simulink model "ieee80211n"  (Simulink 6.0)
settings: Solver=VariableStepDiscrete  StartTime=0.0  StopTime=inf  RelTol=1e-3
PreLoadFcn:
  | load IEEE80211n_init;
values from neighbouring files (symbols this model uses):
  params =     [IEEE80211n_init.mat]    (also in IEEE80211n_settings.m = p)
undefined symbols (not defined in the file or in its folder): magnitude
libraries: commblkintrlv2 x196, dspsigops x143, simulink x136, commdigbbndam2 x98, dspmtrx3 x96, dspsigattribs x69, dspstat3 x38, commutil2 x32, commsequence2 x26, commcnvcod2 x10, dspindex x9, dspmlti3 x8
(part 11 of 12)

== system ieee80211n/training sequence4/Modulator1/Group into OFDM symbols ==
  in1 : Inport  Port=1  LatchInput=off
  in : Inport  Port=2  LatchInput=off
  Assemble Subcarriers : simulink/Math Operations/Matrix Concatenation  numInports=13  catMethod=Vertical
  DC value : Subsystem
      mask Display: disp('Zero DC')
  DC value1 : Subsystem
      mask Display: disp('Zeros, LB')
  DC value2 : Subsystem
      mask Display: disp('Zeros, UB')
  Gain : Gain  Gain=-1  SaturateOnIntegerOverflow=on
  Gain1 : Gain  Gain=-1  SaturateOnIntegerOverflow=on
  Select data blocks : S-Function  AncestorBlock=dspindex/Multiport Selector  FunctionName=sdspmultiportsel  Parameters=rowsOrCols, numOutports, flatIdxVect, flatLenVect, idxErrMode  mask(Multiport Selector){rowsOrCols=Rows, idxCellArray={1:5, 6:18, 19:24, 25:30, 31:43, 44:48}, idxErrMode=Clip Index}
      mask prompts: rowsOrCols "Select:"; idxCellArray "Indices to output:"; idxErrMode "Invalid index:"
      mask help: Output specified rows or columns to one or more output ports. The number of output ports is determined by the number of index vectors, each specified as a separate vector entry in a cell array. Indices are 1-based and need not be unique.
      mask init:
      | [numOutports, flatLenVect, flatIdxVect] = dspblkmultiportsel(idxCellArray);
      mask Help: web(dspbhelp);
      mask StyleString: popup(Rows|Columns),edit,popup(Clip Index|Clip and Warn|Generate Error)
      mask Display: disp(['Select\n' &1]);
  Select pilots : S-Function  AncestorBlock=dspindex/Multiport Selector  FunctionName=sdspmultiportsel  Parameters=rowsOrCols, numOutports, flatIdxVect, flatLenVect, idxErrMode  mask(Multiport Selector){rowsOrCols=Columns, idxCellArray={(1+params.OFDM_LSIG_SymPerFrame):(params.OFDM_LSIG_SymPerFrame+params.OFDM_HTSIG_SymPerFrame)}, idxErrMode=Clip Index}
      mask prompts: rowsOrCols "Select:"; idxCellArray "Indices to output:"; idxErrMode "Invalid index:"
      mask help: Output specified rows or columns to one or more output ports. The number of output ports is determined by the number of index vectors, each specified as a separate vector entry in a cell array. Indices are 1-based and need not be unique.
      mask init:
      | [numOutports, flatLenVect, flatIdxVect] = dspblkmultiportsel(idxCellArray);
      mask Help: web(dspbhelp);
      mask StyleString: popup(Rows|Columns),edit,popup(Clip Index|Clip and Warn|Generate Error)
      mask Display: disp(['Select\n' &1]);
  out : Outport
  wires:
  Select data blocks/1 -> Assemble Subcarriers/2
  Select data blocks/2 -> Assemble Subcarriers/4
  Select data blocks/3 -> Assemble Subcarriers/6
  Select data blocks/4 -> Assemble Subcarriers/8
  Select data blocks/5 -> Assemble Subcarriers/10
  Select data blocks/6 -> Assemble Subcarriers/12
  Gain/1 -> Assemble Subcarriers/11
  in1/1 -> Select pilots/1
  Assemble Subcarriers/1 -> out/1
  DC value/1(out) -> Assemble Subcarriers/7
  in/1 -> Select data blocks/1
  Select pilots/1 -> Gain1/1
  DC value1/1(out) -> Assemble Subcarriers/1
  DC value2/1(out) -> Assemble Subcarriers/13
  Gain1/1 -> Gain/1, Assemble Subcarriers/9, Assemble Subcarriers/5, Assemble Subcarriers/3

== system ieee80211n/training sequence4/Modulator1/Modulator 2 ==
  txdata : Inport  Port=1  LatchInput=off
  Convolutional Encoder1 : commcnvcod2/Convolutional Encoder  trellis=trellisStructure  reset=None
  Gain1 : Gain  SaturateOnIntegerOverflow=on
  General Block Interleaver : commblkintrlv2/General Block Interleaver  elements=interleaverElements
  Matrix Interleaver : commblkintrlv2/Matrix Interleaver  Nrows=interleaverRows  Ncols=interleaverCols
  P2 Puncture : commsequence2/Puncture  punctureVector=punctureVector
  Rectangular QAM Modulator Baseband : commdigbbndam2/Rectangular QAM Modulator Baseband  M=modOrder  InType=Bit  Enc=Gray  PowType=Average Power  MinDist=2  AvgPow=1  PeakPow=1  Ph=0  numSamp=1
  Zero Pad : dspsigops/Zero Pad  padSigAt=End  zpadAlong=Columns  padNumOutRowsSpecMethod=User-specified  numOutRows=bitsPerBlock  padNumOutColsSpecMethod=User-specified  numOutCols=1  trunc_flag=None
      settings: AttributesFormatString=\n
  txsig : Outport
  wires:
  Rectangular QAM Modulator Baseband/1 -> Gain1/1
  Gain1/1 -> txsig/1
  txdata/1 -> Zero Pad/1
  Convolutional Encoder1/1 -> P2 Puncture/1
  Matrix Interleaver/1 -> General Block Interleaver/1
  P2 Puncture/1 -> Matrix Interleaver/1
  General Block Interleaver/1 -> Rectangular QAM Modulator Baseband/1
  Zero Pad/1 -> Convolutional Encoder1/1

== system ieee80211n/training sequence4/Pilots/Unipolar to Bipolar Converter ==
  In1 : Inport  Port=1  LatchInput=off
  Constant : Constant  Orientation=up  Value=M-1
  Gain : Gain  Gain=2
  Polarity : Gain  Gain=pole
  Sum : Sum  Inputs=|+-  InputSameDT=on
  Out1 : Outport
  wires:
  Gain/1 -> Sum/1
  In1/1 -> Gain/1
  Sum/1 -> Polarity/1
  Constant/1 -> Sum/2
  Polarity/1 -> Out1/1

== system ieee80211n/MIMODetection/Channel Estimation/ChannelEst1/Channel estimates ==
  trn : Inport  Port=1  LatchInput=off
  in : Inport  Port=2  LatchInput=off
  Enable Averaging : MultiPortSwitch  Inputs=2  zeroidx=on  SaturateOnIntegerOverflow=on
  Enable Averaging1 : MultiPortSwitch  Inputs=2  zeroidx=on  SaturateOnIntegerOverflow=on
  Frame Status Conversion1 : dspsigattribs/Frame Status Conversion  growRefPort=off  outframe=Frame-based
  Mean : dspstat3/Mean  DialogController=dspDDGCreate  DialogControllerArgs=DataTag3  run=off  reset_popup=None  roundingMode=Floor  overflowMode=off
  Mean1 : dspstat3/Mean  DialogController=dspDDGCreate  DialogControllerArgs=DataTag4  run=off  reset_popup=None  roundingMode=Floor  overflowMode=off
  Nsts > 1 : Constant  Value=params.NSTS > 1
  One sym only (in) : S-Function  AncestorBlock=dspindex/Multiport Selector  FunctionName=sdspmultiportsel  Parameters=rowsOrCols, numOutports, flatIdxVect, flatLenVect, idxErrMode  mask(Multiport Selector){rowsOrCols=Rows, idxCellArray=1, idxErrMode=Clip Index}
      mask prompts: rowsOrCols "Select:"; idxCellArray "Indices to output:"; idxErrMode "Invalid index:"
      mask help: Output specified rows or columns to one or more output ports. The number of output ports is determined by the number of index vectors, each specified as a separate vector entry in a cell array. Indices are 1-based and need not be unique.
      mask init:
      | [numOutports, flatLenVect, flatIdxVect] = dspblkmultiportsel(idxCellArray);
      mask Help: web(dspbhelp);
      mask StyleString: popup(Rows|Columns),edit,popup(Clip Index|Clip and Warn|Generate Error)
      mask Display: disp(['Select\n' &1]);
  One sym only (trn) : S-Function  AncestorBlock=dspindex/Multiport Selector  FunctionName=sdspmultiportsel  Parameters=rowsOrCols, numOutports, flatIdxVect, flatLenVect, idxErrMode  mask(Multiport Selector){rowsOrCols=Rows, idxCellArray=1, idxErrMode=Clip Index}
      mask prompts: rowsOrCols "Select:"; idxCellArray "Indices to output:"; idxErrMode "Invalid index:"
      mask help: Output specified rows or columns to one or more output ports. The number of output ports is determined by the number of index vectors, each specified as a separate vector entry in a cell array. Indices are 1-based and need not be unique.
      mask init:
      | [numOutports, flatLenVect, flatIdxVect] = dspblkmultiportsel(idxCellArray);
      mask Help: web(dspbhelp);
      mask StyleString: popup(Rows|Columns),edit,popup(Clip Index|Clip and Warn|Generate Error)
      mask Display: disp(['Select\n' &1]);
  Product1 : Product  Inputs=**  SaturateOnIntegerOverflow=on
  Product3 : Product  Inputs=/*  SaturateOnIntegerOverflow=on
  Transpose : dspmtrx3/Transpose  Hermitian=off  overflowFlag=on
  Transpose1 : dspmtrx3/Transpose  Hermitian=off  overflowFlag=on
  Transpose2 : dspmtrx3/Transpose  Hermitian=off  overflowFlag=on
  ch est : Outport
  wires:
  trn/1 -> Transpose/1
  Mean/1 -> Enable Averaging/3
  Mean1/1 -> Enable Averaging1/3
  Product3/1 -> Frame Status Conversion1/1
  Transpose/1 -> Product1/1, Product1/2
  Frame Status Conversion1/1 -> Transpose1/1
  Transpose1/1 -> ch est/1
  Transpose2/1 -> Mean1/1, One sym only (in)/1
  Product1/1 -> Mean/1, One sym only (trn)/1
  in/1 -> Transpose2/1
  Enable Averaging/1 -> Product3/1
  Nsts > 1/1 -> Enable Averaging/1, Enable Averaging1/1
  One sym only (in)/1 -> Enable Averaging1/2
  Enable Averaging1/1 -> Product3/2
  One sym only (trn)/1 -> Enable Averaging/2

== system ieee80211n/MIMODetection/Channel Estimation/ChannelEst10/Channel estimates ==
  trn : Inport  Port=1  LatchInput=off
  in : Inport  Port=2  LatchInput=off
  Enable Averaging : MultiPortSwitch  Inputs=2  zeroidx=on  SaturateOnIntegerOverflow=on
  Enable Averaging1 : MultiPortSwitch  Inputs=2  zeroidx=on  SaturateOnIntegerOverflow=on
  Frame Status Conversion1 : dspsigattribs/Frame Status Conversion  growRefPort=off  outframe=Frame-based
  Mean2 : dspstat3/Mean  DialogController=dspDDGCreate  DialogControllerArgs=DataTag5  run=off  reset_popup=None  roundingMode=Floor  overflowMode=off
  Mean3 : dspstat3/Mean  DialogController=dspDDGCreate  DialogControllerArgs=DataTag6  run=off  reset_popup=None  roundingMode=Floor  overflowMode=off
  Nsts > 1 : Constant  Value=params.NSTS > 1
  One sym only (in) : S-Function  AncestorBlock=dspindex/Multiport Selector  FunctionName=sdspmultiportsel  Parameters=rowsOrCols, numOutports, flatIdxVect, flatLenVect, idxErrMode  mask(Multiport Selector){rowsOrCols=Rows, idxCellArray=1, idxErrMode=Clip Index}
      mask prompts: rowsOrCols "Select:"; idxCellArray "Indices to output:"; idxErrMode "Invalid index:"
      mask help: Output specified rows or columns to one or more output ports. The number of output ports is determined by the number of index vectors, each specified as a separate vector entry in a cell array. Indices are 1-based and need not be unique.
      mask init:
      | [numOutports, flatLenVect, flatIdxVect] = dspblkmultiportsel(idxCellArray);
      mask Help: web(dspbhelp);
      mask StyleString: popup(Rows|Columns),edit,popup(Clip Index|Clip and Warn|Generate Error)
      mask Display: disp(['Select\n' &1]);
  One sym only (trn) : S-Function  AncestorBlock=dspindex/Multiport Selector  FunctionName=sdspmultiportsel  Parameters=rowsOrCols, numOutports, flatIdxVect, flatLenVect, idxErrMode  mask(Multiport Selector){rowsOrCols=Rows, idxCellArray=1, idxErrMode=Clip Index}
      mask prompts: rowsOrCols "Select:"; idxCellArray "Indices to output:"; idxErrMode "Invalid index:"
      mask help: Output specified rows or columns to one or more output ports. The number of output ports is determined by the number of index vectors, each specified as a separate vector entry in a cell array. Indices are 1-based and need not be unique.
      mask init:
      | [numOutports, flatLenVect, flatIdxVect] = dspblkmultiportsel(idxCellArray);
      mask Help: web(dspbhelp);
      mask StyleString: popup(Rows|Columns),edit,popup(Clip Index|Clip and Warn|Generate Error)
      mask Display: disp(['Select\n' &1]);
  Product2 : Product  Inputs=**  SaturateOnIntegerOverflow=on
  Product4 : Product  Inputs=/*  SaturateOnIntegerOverflow=on
  Transpose : dspmtrx3/Transpose  Hermitian=off  overflowFlag=on
  Transpose1 : dspmtrx3/Transpose  Hermitian=off  overflowFlag=on
  Transpose2 : dspmtrx3/Transpose  Hermitian=off  overflowFlag=on
  ch est : Outport
  wires:
  trn/1 -> Transpose/1
  Product4/1 -> Frame Status Conversion1/1
  Frame Status Conversion1/1 -> Transpose1/1
  Transpose1/1 -> ch est/1
  in/1 -> Transpose2/1
  Mean2/1 -> Enable Averaging/3
  Mean3/1 -> Enable Averaging1/3
  Transpose/1 -> Product2/1, Product2/2
  Transpose2/1 -> Mean3/1, One sym only (in)/1
  Product2/1 -> Mean2/1, One sym only (trn)/1
  Enable Averaging/1 -> Product4/1
  Nsts > 1/1 -> Enable Averaging/1, Enable Averaging1/1
  One sym only (in)/1 -> Enable Averaging1/2
  Enable Averaging1/1 -> Product4/2
  One sym only (trn)/1 -> Enable Averaging/2

== system ieee80211n/MIMODetection/Channel Estimation/ChannelEst11/Channel estimates ==
  trn : Inport  Port=1  LatchInput=off
  in : Inport  Port=2  LatchInput=off
  Enable Averaging : MultiPortSwitch  Inputs=2  zeroidx=on  SaturateOnIntegerOverflow=on
  Enable Averaging1 : MultiPortSwitch  Inputs=2  zeroidx=on  SaturateOnIntegerOverflow=on
  Frame Status Conversion1 : dspsigattribs/Frame Status Conversion  growRefPort=off  outframe=Frame-based
  Mean2 : dspstat3/Mean  DialogController=dspDDGCreate  DialogControllerArgs=DataTag7  run=off  reset_popup=None  roundingMode=Floor  overflowMode=off
  Mean3 : dspstat3/Mean  DialogController=dspDDGCreate  DialogControllerArgs=DataTag8  run=off  reset_popup=None  roundingMode=Floor  overflowMode=off
  Nsts > 1 : Constant  Value=params.NSTS > 1
  One sym only (in) : S-Function  AncestorBlock=dspindex/Multiport Selector  FunctionName=sdspmultiportsel  Parameters=rowsOrCols, numOutports, flatIdxVect, flatLenVect, idxErrMode  mask(Multiport Selector){rowsOrCols=Rows, idxCellArray=1, idxErrMode=Clip Index}
      mask prompts: rowsOrCols "Select:"; idxCellArray "Indices to output:"; idxErrMode "Invalid index:"
      mask help: Output specified rows or columns to one or more output ports. The number of output ports is determined by the number of index vectors, each specified as a separate vector entry in a cell array. Indices are 1-based and need not be unique.
      mask init:
      | [numOutports, flatLenVect, flatIdxVect] = dspblkmultiportsel(idxCellArray);
      mask Help: web(dspbhelp);
      mask StyleString: popup(Rows|Columns),edit,popup(Clip Index|Clip and Warn|Generate Error)
      mask Display: disp(['Select\n' &1]);
  One sym only (trn) : S-Function  AncestorBlock=dspindex/Multiport Selector  FunctionName=sdspmultiportsel  Parameters=rowsOrCols, numOutports, flatIdxVect, flatLenVect, idxErrMode  mask(Multiport Selector){rowsOrCols=Rows, idxCellArray=1, idxErrMode=Clip Index}
      mask prompts: rowsOrCols "Select:"; idxCellArray "Indices to output:"; idxErrMode "Invalid index:"
      mask help: Output specified rows or columns to one or more output ports. The number of output ports is determined by the number of index vectors, each specified as a separate vector entry in a cell array. Indices are 1-based and need not be unique.
      mask init:
      | [numOutports, flatLenVect, flatIdxVect] = dspblkmultiportsel(idxCellArray);
      mask Help: web(dspbhelp);
      mask StyleString: popup(Rows|Columns),edit,popup(Clip Index|Clip and Warn|Generate Error)
      mask Display: disp(['Select\n' &1]);
  Product2 : Product  Inputs=**  SaturateOnIntegerOverflow=on
  Product4 : Product  Inputs=/*  SaturateOnIntegerOverflow=on
  Transpose : dspmtrx3/Transpose  Hermitian=off  overflowFlag=on
  Transpose1 : dspmtrx3/Transpose  Hermitian=off  overflowFlag=on
  Transpose2 : dspmtrx3/Transpose  Hermitian=off  overflowFlag=on
  ch est : Outport
  wires:
  trn/1 -> Transpose/1
  Product4/1 -> Frame Status Conversion1/1
  Frame Status Conversion1/1 -> Transpose1/1
  Transpose1/1 -> ch est/1
  in/1 -> Transpose2/1
  Mean2/1 -> Enable Averaging/3
  Mean3/1 -> Enable Averaging1/3
  Transpose/1 -> Product2/1, Product2/2
  Transpose2/1 -> Mean3/1, One sym only (in)/1
  Product2/1 -> Mean2/1, One sym only (trn)/1
  Enable Averaging/1 -> Product4/1
  Nsts > 1/1 -> Enable Averaging/1, Enable Averaging1/1
  One sym only (in)/1 -> Enable Averaging1/2
  Enable Averaging1/1 -> Product4/2
  One sym only (trn)/1 -> Enable Averaging/2

== system ieee80211n/MIMODetection/Channel Estimation/ChannelEst12/Channel estimates ==
  trn : Inport  Port=1  LatchInput=off
  in : Inport  Port=2  LatchInput=off
  Enable Averaging : MultiPortSwitch  Inputs=2  zeroidx=on  SaturateOnIntegerOverflow=on
  Enable Averaging1 : MultiPortSwitch  Inputs=2  zeroidx=on  SaturateOnIntegerOverflow=on
  Frame Status Conversion1 : dspsigattribs/Frame Status Conversion  growRefPort=off  outframe=Frame-based
  Mean2 : dspstat3/Mean  DialogController=dspDDGCreate  DialogControllerArgs=DataTag9  run=off  reset_popup=None  roundingMode=Floor  overflowMode=off
  Mean3 : dspstat3/Mean  DialogController=dspDDGCreate  DialogControllerArgs=DataTag10  run=off  reset_popup=None  roundingMode=Floor  overflowMode=off
  Nsts > 1 : Constant  Value=params.NSTS > 1
  One sym only (in) : S-Function  AncestorBlock=dspindex/Multiport Selector  FunctionName=sdspmultiportsel  Parameters=rowsOrCols, numOutports, flatIdxVect, flatLenVect, idxErrMode  mask(Multiport Selector){rowsOrCols=Rows, idxCellArray=1, idxErrMode=Clip Index}
      mask prompts: rowsOrCols "Select:"; idxCellArray "Indices to output:"; idxErrMode "Invalid index:"
      mask help: Output specified rows or columns to one or more output ports. The number of output ports is determined by the number of index vectors, each specified as a separate vector entry in a cell array. Indices are 1-based and need not be unique.
      mask init:
      | [numOutports, flatLenVect, flatIdxVect] = dspblkmultiportsel(idxCellArray);
      mask Help: web(dspbhelp);
      mask StyleString: popup(Rows|Columns),edit,popup(Clip Index|Clip and Warn|Generate Error)
      mask Display: disp(['Select\n' &1]);
  One sym only (trn) : S-Function  AncestorBlock=dspindex/Multiport Selector  FunctionName=sdspmultiportsel  Parameters=rowsOrCols, numOutports, flatIdxVect, flatLenVect, idxErrMode  mask(Multiport Selector){rowsOrCols=Rows, idxCellArray=1, idxErrMode=Clip Index}
      mask prompts: rowsOrCols "Select:"; idxCellArray "Indices to output:"; idxErrMode "Invalid index:"
      mask help: Output specified rows or columns to one or more output ports. The number of output ports is determined by the number of index vectors, each specified as a separate vector entry in a cell array. Indices are 1-based and need not be unique.
      mask init:
      | [numOutports, flatLenVect, flatIdxVect] = dspblkmultiportsel(idxCellArray);
      mask Help: web(dspbhelp);
      mask StyleString: popup(Rows|Columns),edit,popup(Clip Index|Clip and Warn|Generate Error)
      mask Display: disp(['Select\n' &1]);
  Product2 : Product  Inputs=**  SaturateOnIntegerOverflow=on
  Product4 : Product  Inputs=/*  SaturateOnIntegerOverflow=on
  Transpose : dspmtrx3/Transpose  Hermitian=off  overflowFlag=on
  Transpose1 : dspmtrx3/Transpose  Hermitian=off  overflowFlag=on
  Transpose2 : dspmtrx3/Transpose  Hermitian=off  overflowFlag=on
  ch est : Outport
  wires:
  trn/1 -> Transpose/1
  Product4/1 -> Frame Status Conversion1/1
  Frame Status Conversion1/1 -> Transpose1/1
  Transpose1/1 -> ch est/1
  in/1 -> Transpose2/1
  Mean2/1 -> Enable Averaging/3
  Mean3/1 -> Enable Averaging1/3
  Transpose/1 -> Product2/1, Product2/2
  Transpose2/1 -> Mean3/1, One sym only (in)/1
  Product2/1 -> Mean2/1, One sym only (trn)/1
  Enable Averaging/1 -> Product4/1
  Nsts > 1/1 -> Enable Averaging/1, Enable Averaging1/1
  One sym only (in)/1 -> Enable Averaging1/2
  Enable Averaging1/1 -> Product4/2
  One sym only (trn)/1 -> Enable Averaging/2

== system ieee80211n/MIMODetection/Channel Estimation/ChannelEst13/Channel estimates ==
  trn : Inport  Port=1  LatchInput=off
  in : Inport  Port=2  LatchInput=off
  Enable Averaging : MultiPortSwitch  Inputs=2  zeroidx=on  SaturateOnIntegerOverflow=on
  Enable Averaging1 : MultiPortSwitch  Inputs=2  zeroidx=on  SaturateOnIntegerOverflow=on
  Frame Status Conversion1 : dspsigattribs/Frame Status Conversion  growRefPort=off  outframe=Frame-based
  Mean2 : dspstat3/Mean  DialogController=dspDDGCreate  DialogControllerArgs=DataTag11  run=off  reset_popup=None  roundingMode=Floor  overflowMode=off
  Mean3 : dspstat3/Mean  DialogController=dspDDGCreate  DialogControllerArgs=DataTag12  run=off  reset_popup=None  roundingMode=Floor  overflowMode=off
  Nsts > 1 : Constant  Value=params.NSTS > 1
  One sym only (in) : S-Function  AncestorBlock=dspindex/Multiport Selector  FunctionName=sdspmultiportsel  Parameters=rowsOrCols, numOutports, flatIdxVect, flatLenVect, idxErrMode  mask(Multiport Selector){rowsOrCols=Rows, idxCellArray=1, idxErrMode=Clip Index}
      mask prompts: rowsOrCols "Select:"; idxCellArray "Indices to output:"; idxErrMode "Invalid index:"
      mask help: Output specified rows or columns to one or more output ports. The number of output ports is determined by the number of index vectors, each specified as a separate vector entry in a cell array. Indices are 1-based and need not be unique.
      mask init:
      | [numOutports, flatLenVect, flatIdxVect] = dspblkmultiportsel(idxCellArray);
      mask Help: web(dspbhelp);
      mask StyleString: popup(Rows|Columns),edit,popup(Clip Index|Clip and Warn|Generate Error)
      mask Display: disp(['Select\n' &1]);
  One sym only (trn) : S-Function  AncestorBlock=dspindex/Multiport Selector  FunctionName=sdspmultiportsel  Parameters=rowsOrCols, numOutports, flatIdxVect, flatLenVect, idxErrMode  mask(Multiport Selector){rowsOrCols=Rows, idxCellArray=1, idxErrMode=Clip Index}
      mask prompts: rowsOrCols "Select:"; idxCellArray "Indices to output:"; idxErrMode "Invalid index:"
      mask help: Output specified rows or columns to one or more output ports. The number of output ports is determined by the number of index vectors, each specified as a separate vector entry in a cell array. Indices are 1-based and need not be unique.
      mask init:
      | [numOutports, flatLenVect, flatIdxVect] = dspblkmultiportsel(idxCellArray);
      mask Help: web(dspbhelp);
      mask StyleString: popup(Rows|Columns),edit,popup(Clip Index|Clip and Warn|Generate Error)
      mask Display: disp(['Select\n' &1]);
  Product2 : Product  Inputs=**  SaturateOnIntegerOverflow=on
  Product4 : Product  Inputs=/*  SaturateOnIntegerOverflow=on
  Transpose : dspmtrx3/Transpose  Hermitian=off  overflowFlag=on
  Transpose1 : dspmtrx3/Transpose  Hermitian=off  overflowFlag=on
  Transpose2 : dspmtrx3/Transpose  Hermitian=off  overflowFlag=on
  ch est : Outport
  wires:
  trn/1 -> Transpose/1
  Product4/1 -> Frame Status Conversion1/1
  Frame Status Conversion1/1 -> Transpose1/1
  Transpose1/1 -> ch est/1
  in/1 -> Transpose2/1
  Mean2/1 -> Enable Averaging/3
  Mean3/1 -> Enable Averaging1/3
  Transpose/1 -> Product2/1, Product2/2
  Transpose2/1 -> Mean3/1, One sym only (in)/1
  Product2/1 -> Mean2/1, One sym only (trn)/1
  Enable Averaging/1 -> Product4/1
  Nsts > 1/1 -> Enable Averaging/1, Enable Averaging1/1
  One sym only (in)/1 -> Enable Averaging1/2
  Enable Averaging1/1 -> Product4/2
  One sym only (trn)/1 -> Enable Averaging/2

== system ieee80211n/MIMODetection/Channel Estimation/ChannelEst14/Channel estimates ==
  trn : Inport  Port=1  LatchInput=off
  in : Inport  Port=2  LatchInput=off
  Enable Averaging : MultiPortSwitch  Inputs=2  zeroidx=on  SaturateOnIntegerOverflow=on
  Enable Averaging1 : MultiPortSwitch  Inputs=2  zeroidx=on  SaturateOnIntegerOverflow=on
  Frame Status Conversion1 : dspsigattribs/Frame Status Conversion  growRefPort=off  outframe=Frame-based
  Mean2 : dspstat3/Mean  DialogController=dspDDGCreate  DialogControllerArgs=DataTag13  run=off  reset_popup=None  roundingMode=Floor  overflowMode=off
  Mean3 : dspstat3/Mean  DialogController=dspDDGCreate  DialogControllerArgs=DataTag14  run=off  reset_popup=None  roundingMode=Floor  overflowMode=off
  Nsts > 1 : Constant  Value=params.NSTS > 1
  One sym only (in) : S-Function  AncestorBlock=dspindex/Multiport Selector  FunctionName=sdspmultiportsel  Parameters=rowsOrCols, numOutports, flatIdxVect, flatLenVect, idxErrMode  mask(Multiport Selector){rowsOrCols=Rows, idxCellArray=1, idxErrMode=Clip Index}
      mask prompts: rowsOrCols "Select:"; idxCellArray "Indices to output:"; idxErrMode "Invalid index:"
      mask help: Output specified rows or columns to one or more output ports. The number of output ports is determined by the number of index vectors, each specified as a separate vector entry in a cell array. Indices are 1-based and need not be unique.
      mask init:
      | [numOutports, flatLenVect, flatIdxVect] = dspblkmultiportsel(idxCellArray);
      mask Help: web(dspbhelp);
      mask StyleString: popup(Rows|Columns),edit,popup(Clip Index|Clip and Warn|Generate Error)
      mask Display: disp(['Select\n' &1]);
  One sym only (trn) : S-Function  AncestorBlock=dspindex/Multiport Selector  FunctionName=sdspmultiportsel  Parameters=rowsOrCols, numOutports, flatIdxVect, flatLenVect, idxErrMode  mask(Multiport Selector){rowsOrCols=Rows, idxCellArray=1, idxErrMode=Clip Index}
      mask prompts: rowsOrCols "Select:"; idxCellArray "Indices to output:"; idxErrMode "Invalid index:"
      mask help: Output specified rows or columns to one or more output ports. The number of output ports is determined by the number of index vectors, each specified as a separate vector entry in a cell array. Indices are 1-based and need not be unique.
      mask init:
      | [numOutports, flatLenVect, flatIdxVect] = dspblkmultiportsel(idxCellArray);
      mask Help: web(dspbhelp);
      mask StyleString: popup(Rows|Columns),edit,popup(Clip Index|Clip and Warn|Generate Error)
      mask Display: disp(['Select\n' &1]);
  Product2 : Product  Inputs=**  SaturateOnIntegerOverflow=on
  Product4 : Product  Inputs=/*  SaturateOnIntegerOverflow=on
  Transpose : dspmtrx3/Transpose  Hermitian=off  overflowFlag=on
  Transpose1 : dspmtrx3/Transpose  Hermitian=off  overflowFlag=on
  Transpose2 : dspmtrx3/Transpose  Hermitian=off  overflowFlag=on
  ch est : Outport
  wires:
  trn/1 -> Transpose/1
  Product4/1 -> Frame Status Conversion1/1
  Frame Status Conversion1/1 -> Transpose1/1
  Transpose1/1 -> ch est/1
  in/1 -> Transpose2/1
  Mean2/1 -> Enable Averaging/3
  Mean3/1 -> Enable Averaging1/3
  Transpose/1 -> Product2/1, Product2/2
  Transpose2/1 -> Mean3/1, One sym only (in)/1
  Product2/1 -> Mean2/1, One sym only (trn)/1
  Enable Averaging/1 -> Product4/1
  Nsts > 1/1 -> Enable Averaging/1, Enable Averaging1/1
  One sym only (in)/1 -> Enable Averaging1/2
  Enable Averaging1/1 -> Product4/2
  One sym only (trn)/1 -> Enable Averaging/2

== system ieee80211n/MIMODetection/Channel Estimation/ChannelEst15/Channel estimates ==
  trn : Inport  Port=1  LatchInput=off
  in : Inport  Port=2  LatchInput=off
  Enable Averaging : MultiPortSwitch  Inputs=2  zeroidx=on  SaturateOnIntegerOverflow=on
  Enable Averaging1 : MultiPortSwitch  Inputs=2  zeroidx=on  SaturateOnIntegerOverflow=on
  Frame Status Conversion1 : dspsigattribs/Frame Status Conversion  growRefPort=off  outframe=Frame-based
  Mean2 : dspstat3/Mean  DialogController=dspDDGCreate  DialogControllerArgs=DataTag15  run=off  reset_popup=None  roundingMode=Floor  overflowMode=off
  Mean3 : dspstat3/Mean  DialogController=dspDDGCreate  DialogControllerArgs=DataTag16  run=off  reset_popup=None  roundingMode=Floor  overflowMode=off
  Nsts > 1 : Constant  Value=params.NSTS > 1
  One sym only (in) : S-Function  AncestorBlock=dspindex/Multiport Selector  FunctionName=sdspmultiportsel  Parameters=rowsOrCols, numOutports, flatIdxVect, flatLenVect, idxErrMode  mask(Multiport Selector){rowsOrCols=Rows, idxCellArray=1, idxErrMode=Clip Index}
      mask prompts: rowsOrCols "Select:"; idxCellArray "Indices to output:"; idxErrMode "Invalid index:"
      mask help: Output specified rows or columns to one or more output ports. The number of output ports is determined by the number of index vectors, each specified as a separate vector entry in a cell array. Indices are 1-based and need not be unique.
      mask init:
      | [numOutports, flatLenVect, flatIdxVect] = dspblkmultiportsel(idxCellArray);
      mask Help: web(dspbhelp);
      mask StyleString: popup(Rows|Columns),edit,popup(Clip Index|Clip and Warn|Generate Error)
      mask Display: disp(['Select\n' &1]);
  One sym only (trn) : S-Function  AncestorBlock=dspindex/Multiport Selector  FunctionName=sdspmultiportsel  Parameters=rowsOrCols, numOutports, flatIdxVect, flatLenVect, idxErrMode  mask(Multiport Selector){rowsOrCols=Rows, idxCellArray=1, idxErrMode=Clip Index}
      mask prompts: rowsOrCols "Select:"; idxCellArray "Indices to output:"; idxErrMode "Invalid index:"
      mask help: Output specified rows or columns to one or more output ports. The number of output ports is determined by the number of index vectors, each specified as a separate vector entry in a cell array. Indices are 1-based and need not be unique.
      mask init:
      | [numOutports, flatLenVect, flatIdxVect] = dspblkmultiportsel(idxCellArray);
      mask Help: web(dspbhelp);
      mask StyleString: popup(Rows|Columns),edit,popup(Clip Index|Clip and Warn|Generate Error)
      mask Display: disp(['Select\n' &1]);
  Product2 : Product  Inputs=**  SaturateOnIntegerOverflow=on
  Product4 : Product  Inputs=/*  SaturateOnIntegerOverflow=on
  Transpose : dspmtrx3/Transpose  Hermitian=off  overflowFlag=on
  Transpose1 : dspmtrx3/Transpose  Hermitian=off  overflowFlag=on
  Transpose2 : dspmtrx3/Transpose  Hermitian=off  overflowFlag=on
  ch est : Outport
  wires:
  trn/1 -> Transpose/1
  Product4/1 -> Frame Status Conversion1/1
  Frame Status Conversion1/1 -> Transpose1/1
  Transpose1/1 -> ch est/1
  in/1 -> Transpose2/1
  Mean2/1 -> Enable Averaging/3
  Mean3/1 -> Enable Averaging1/3
  Transpose/1 -> Product2/1, Product2/2
  Transpose2/1 -> Mean3/1, One sym only (in)/1
  Product2/1 -> Mean2/1, One sym only (trn)/1
  Enable Averaging/1 -> Product4/1
  Nsts > 1/1 -> Enable Averaging/1, Enable Averaging1/1
  One sym only (in)/1 -> Enable Averaging1/2
  Enable Averaging1/1 -> Product4/2
  One sym only (trn)/1 -> Enable Averaging/2

== system ieee80211n/MIMODetection/Channel Estimation/ChannelEst16/Channel estimates ==
  trn : Inport  Port=1  LatchInput=off
  in : Inport  Port=2  LatchInput=off
  Enable Averaging : MultiPortSwitch  Inputs=2  zeroidx=on  SaturateOnIntegerOverflow=on
  Enable Averaging1 : MultiPortSwitch  Inputs=2  zeroidx=on  SaturateOnIntegerOverflow=on
  Frame Status Conversion1 : dspsigattribs/Frame Status Conversion  growRefPort=off  outframe=Frame-based
  Mean2 : dspstat3/Mean  DialogController=dspDDGCreate  DialogControllerArgs=DataTag17  run=off  reset_popup=None  roundingMode=Floor  overflowMode=off
  Mean3 : dspstat3/Mean  DialogController=dspDDGCreate  DialogControllerArgs=DataTag18  run=off  reset_popup=None  roundingMode=Floor  overflowMode=off
  Nsts > 1 : Constant  Value=params.NSTS > 1
  One sym only (in) : S-Function  AncestorBlock=dspindex/Multiport Selector  FunctionName=sdspmultiportsel  Parameters=rowsOrCols, numOutports, flatIdxVect, flatLenVect, idxErrMode  mask(Multiport Selector){rowsOrCols=Rows, idxCellArray=1, idxErrMode=Clip Index}
      mask prompts: rowsOrCols "Select:"; idxCellArray "Indices to output:"; idxErrMode "Invalid index:"
      mask help: Output specified rows or columns to one or more output ports. The number of output ports is determined by the number of index vectors, each specified as a separate vector entry in a cell array. Indices are 1-based and need not be unique.
      mask init:
      | [numOutports, flatLenVect, flatIdxVect] = dspblkmultiportsel(idxCellArray);
      mask Help: web(dspbhelp);
      mask StyleString: popup(Rows|Columns),edit,popup(Clip Index|Clip and Warn|Generate Error)
      mask Display: disp(['Select\n' &1]);
  One sym only (trn) : S-Function  AncestorBlock=dspindex/Multiport Selector  FunctionName=sdspmultiportsel  Parameters=rowsOrCols, numOutports, flatIdxVect, flatLenVect, idxErrMode  mask(Multiport Selector){rowsOrCols=Rows, idxCellArray=1, idxErrMode=Clip Index}
      mask prompts: rowsOrCols "Select:"; idxCellArray "Indices to output:"; idxErrMode "Invalid index:"
      mask help: Output specified rows or columns to one or more output ports. The number of output ports is determined by the number of index vectors, each specified as a separate vector entry in a cell array. Indices are 1-based and need not be unique.
      mask init:
      | [numOutports, flatLenVect, flatIdxVect] = dspblkmultiportsel(idxCellArray);
      mask Help: web(dspbhelp);
      mask StyleString: popup(Rows|Columns),edit,popup(Clip Index|Clip and Warn|Generate Error)
      mask Display: disp(['Select\n' &1]);
  Product2 : Product  Inputs=**  SaturateOnIntegerOverflow=on
  Product4 : Product  Inputs=/*  SaturateOnIntegerOverflow=on
  Transpose : dspmtrx3/Transpose  Hermitian=off  overflowFlag=on
  Transpose1 : dspmtrx3/Transpose  Hermitian=off  overflowFlag=on
  Transpose2 : dspmtrx3/Transpose  Hermitian=off  overflowFlag=on
  ch est : Outport
  wires:
  trn/1 -> Transpose/1
  Product4/1 -> Frame Status Conversion1/1
  Frame Status Conversion1/1 -> Transpose1/1
  Transpose1/1 -> ch est/1
  in/1 -> Transpose2/1
  Mean2/1 -> Enable Averaging/3
  Mean3/1 -> Enable Averaging1/3
  Transpose/1 -> Product2/1, Product2/2
  Transpose2/1 -> Mean3/1, One sym only (in)/1
  Product2/1 -> Mean2/1, One sym only (trn)/1
  Enable Averaging/1 -> Product4/1
  Nsts > 1/1 -> Enable Averaging/1, Enable Averaging1/1
  One sym only (in)/1 -> Enable Averaging1/2
  Enable Averaging1/1 -> Product4/2
  One sym only (trn)/1 -> Enable Averaging/2

== system ieee80211n/MIMODetection/Channel Estimation/ChannelEst2/Channel estimates ==
  trn : Inport  Port=1  LatchInput=off
  in : Inport  Port=2  LatchInput=off
  Enable Averaging : MultiPortSwitch  Inputs=2  zeroidx=on  SaturateOnIntegerOverflow=on
  Enable Averaging1 : MultiPortSwitch  Inputs=2  zeroidx=on  SaturateOnIntegerOverflow=on
  Frame Status Conversion1 : dspsigattribs/Frame Status Conversion  growRefPort=off  outframe=Frame-based
  Mean : dspstat3/Mean  DialogController=dspDDGCreate  DialogControllerArgs=DataTag19  run=off  reset_popup=None  roundingMode=Floor  overflowMode=off
  Mean1 : dspstat3/Mean  DialogController=dspDDGCreate  DialogControllerArgs=DataTag20  run=off  reset_popup=None  roundingMode=Floor  overflowMode=off
  Nsts > 1 : Constant  Value=params.NSTS > 1
  One sym only (in) : S-Function  AncestorBlock=dspindex/Multiport Selector  FunctionName=sdspmultiportsel  Parameters=rowsOrCols, numOutports, flatIdxVect, flatLenVect, idxErrMode  mask(Multiport Selector){rowsOrCols=Rows, idxCellArray=1, idxErrMode=Clip Index}
      mask prompts: rowsOrCols "Select:"; idxCellArray "Indices to output:"; idxErrMode "Invalid index:"
      mask help: Output specified rows or columns to one or more output ports. The number of output ports is determined by the number of index vectors, each specified as a separate vector entry in a cell array. Indices are 1-based and need not be unique.
      mask init:
      | [numOutports, flatLenVect, flatIdxVect] = dspblkmultiportsel(idxCellArray);
      mask Help: web(dspbhelp);
      mask StyleString: popup(Rows|Columns),edit,popup(Clip Index|Clip and Warn|Generate Error)
      mask Display: disp(['Select\n' &1]);
  One sym only (trn) : S-Function  AncestorBlock=dspindex/Multiport Selector  FunctionName=sdspmultiportsel  Parameters=rowsOrCols, numOutports, flatIdxVect, flatLenVect, idxErrMode  mask(Multiport Selector){rowsOrCols=Rows, idxCellArray=1, idxErrMode=Clip Index}
      mask prompts: rowsOrCols "Select:"; idxCellArray "Indices to output:"; idxErrMode "Invalid index:"
      mask help: Output specified rows or columns to one or more output ports. The number of output ports is determined by the number of index vectors, each specified as a separate vector entry in a cell array. Indices are 1-based and need not be unique.
      mask init:
      | [numOutports, flatLenVect, flatIdxVect] = dspblkmultiportsel(idxCellArray);
      mask Help: web(dspbhelp);
      mask StyleString: popup(Rows|Columns),edit,popup(Clip Index|Clip and Warn|Generate Error)
      mask Display: disp(['Select\n' &1]);
  Product1 : Product  Inputs=**  SaturateOnIntegerOverflow=on
  Product3 : Product  Inputs=/*  SaturateOnIntegerOverflow=on
  Transpose : dspmtrx3/Transpose  Hermitian=off  overflowFlag=on
  Transpose1 : dspmtrx3/Transpose  Hermitian=off  overflowFlag=on
  Transpose2 : dspmtrx3/Transpose  Hermitian=off  overflowFlag=on
  ch est : Outport
  wires:
  trn/1 -> Transpose/1
  Frame Status Conversion1/1 -> Transpose1/1
  Transpose1/1 -> ch est/1
  in/1 -> Transpose2/1
  Mean/1 -> Enable Averaging/3
  Mean1/1 -> Enable Averaging1/3
  Product3/1 -> Frame Status Conversion1/1
  Transpose/1 -> Product1/1, Product1/2
  Transpose2/1 -> Mean1/1, One sym only (in)/1
  Product1/1 -> Mean/1, One sym only (trn)/1
  Enable Averaging/1 -> Product3/1
  Nsts > 1/1 -> Enable Averaging/1, Enable Averaging1/1
  One sym only (in)/1 -> Enable Averaging1/2
  Enable Averaging1/1 -> Product3/2
  One sym only (trn)/1 -> Enable Averaging/2

== system ieee80211n/MIMODetection/Channel Estimation/ChannelEst3/Channel estimates ==
  trn : Inport  Port=1  LatchInput=off
  in : Inport  Port=2  LatchInput=off
  Enable Averaging : MultiPortSwitch  Inputs=2  zeroidx=on  SaturateOnIntegerOverflow=on
  Enable Averaging1 : MultiPortSwitch  Inputs=2  zeroidx=on  SaturateOnIntegerOverflow=on
  Frame Status Conversion1 : dspsigattribs/Frame Status Conversion  growRefPort=off  outframe=Frame-based
  Mean2 : dspstat3/Mean  DialogController=dspDDGCreate  DialogControllerArgs=DataTag21  run=off  reset_popup=None  roundingMode=Floor  overflowMode=off
  Mean3 : dspstat3/Mean  DialogController=dspDDGCreate  DialogControllerArgs=DataTag22  run=off  reset_popup=None  roundingMode=Floor  overflowMode=off
  Nsts > 1 : Constant  Value=params.NSTS > 1
  One sym only (in) : S-Function  AncestorBlock=dspindex/Multiport Selector  FunctionName=sdspmultiportsel  Parameters=rowsOrCols, numOutports, flatIdxVect, flatLenVect, idxErrMode  mask(Multiport Selector){rowsOrCols=Rows, idxCellArray=1, idxErrMode=Clip Index}
      mask prompts: rowsOrCols "Select:"; idxCellArray "Indices to output:"; idxErrMode "Invalid index:"
      mask help: Output specified rows or columns to one or more output ports. The number of output ports is determined by the number of index vectors, each specified as a separate vector entry in a cell array. Indices are 1-based and need not be unique.
      mask init:
      | [numOutports, flatLenVect, flatIdxVect] = dspblkmultiportsel(idxCellArray);
      mask Help: web(dspbhelp);
      mask StyleString: popup(Rows|Columns),edit,popup(Clip Index|Clip and Warn|Generate Error)
      mask Display: disp(['Select\n' &1]);
  One sym only (trn) : S-Function  AncestorBlock=dspindex/Multiport Selector  FunctionName=sdspmultiportsel  Parameters=rowsOrCols, numOutports, flatIdxVect, flatLenVect, idxErrMode  mask(Multiport Selector){rowsOrCols=Rows, idxCellArray=1, idxErrMode=Clip Index}
      mask prompts: rowsOrCols "Select:"; idxCellArray "Indices to output:"; idxErrMode "Invalid index:"
      mask help: Output specified rows or columns to one or more output ports. The number of output ports is determined by the number of index vectors, each specified as a separate vector entry in a cell array. Indices are 1-based and need not be unique.
      mask init:
      | [numOutports, flatLenVect, flatIdxVect] = dspblkmultiportsel(idxCellArray);
      mask Help: web(dspbhelp);
      mask StyleString: popup(Rows|Columns),edit,popup(Clip Index|Clip and Warn|Generate Error)
      mask Display: disp(['Select\n' &1]);
  Product2 : Product  Inputs=**  SaturateOnIntegerOverflow=on
  Product4 : Product  Inputs=/*  SaturateOnIntegerOverflow=on
  Transpose : dspmtrx3/Transpose  Hermitian=off  overflowFlag=on
  Transpose1 : dspmtrx3/Transpose  Hermitian=off  overflowFlag=on
  Transpose2 : dspmtrx3/Transpose  Hermitian=off  overflowFlag=on
  ch est : Outport
  wires:
  trn/1 -> Transpose/1
  Product4/1 -> Frame Status Conversion1/1
  Frame Status Conversion1/1 -> Transpose1/1
  Transpose1/1 -> ch est/1
  in/1 -> Transpose2/1
  Mean2/1 -> Enable Averaging/3
  Mean3/1 -> Enable Averaging1/3
  Transpose/1 -> Product2/1, Product2/2
  Transpose2/1 -> Mean3/1, One sym only (in)/1
  Product2/1 -> Mean2/1, One sym only (trn)/1
  Enable Averaging/1 -> Product4/1
  Nsts > 1/1 -> Enable Averaging/1, Enable Averaging1/1
  One sym only (in)/1 -> Enable Averaging1/2
  Enable Averaging1/1 -> Product4/2
  One sym only (trn)/1 -> Enable Averaging/2

== system ieee80211n/MIMODetection/Channel Estimation/ChannelEst4/Channel estimates ==
  trn : Inport  Port=1  LatchInput=off
  in : Inport  Port=2  LatchInput=off
  Enable Averaging : MultiPortSwitch  Inputs=2  zeroidx=on  SaturateOnIntegerOverflow=on
  Enable Averaging1 : MultiPortSwitch  Inputs=2  zeroidx=on  SaturateOnIntegerOverflow=on
  Frame Status Conversion1 : dspsigattribs/Frame Status Conversion  growRefPort=off  outframe=Frame-based
  Mean2 : dspstat3/Mean  DialogController=dspDDGCreate  DialogControllerArgs=DataTag23  run=off  reset_popup=None  roundingMode=Floor  overflowMode=off
  Mean3 : dspstat3/Mean  DialogController=dspDDGCreate  DialogControllerArgs=DataTag24  run=off  reset_popup=None  roundingMode=Floor  overflowMode=off
  Nsts > 1 : Constant  Value=params.NSTS > 1
  One sym only (in) : S-Function  AncestorBlock=dspindex/Multiport Selector  FunctionName=sdspmultiportsel  Parameters=rowsOrCols, numOutports, flatIdxVect, flatLenVect, idxErrMode  mask(Multiport Selector){rowsOrCols=Rows, idxCellArray=1, idxErrMode=Clip Index}
      mask prompts: rowsOrCols "Select:"; idxCellArray "Indices to output:"; idxErrMode "Invalid index:"
      mask help: Output specified rows or columns to one or more output ports. The number of output ports is determined by the number of index vectors, each specified as a separate vector entry in a cell array. Indices are 1-based and need not be unique.
      mask init:
      | [numOutports, flatLenVect, flatIdxVect] = dspblkmultiportsel(idxCellArray);
      mask Help: web(dspbhelp);
      mask StyleString: popup(Rows|Columns),edit,popup(Clip Index|Clip and Warn|Generate Error)
      mask Display: disp(['Select\n' &1]);
  One sym only (trn) : S-Function  AncestorBlock=dspindex/Multiport Selector  FunctionName=sdspmultiportsel  Parameters=rowsOrCols, numOutports, flatIdxVect, flatLenVect, idxErrMode  mask(Multiport Selector){rowsOrCols=Rows, idxCellArray=1, idxErrMode=Clip Index}
      mask prompts: rowsOrCols "Select:"; idxCellArray "Indices to output:"; idxErrMode "Invalid index:"
      mask help: Output specified rows or columns to one or more output ports. The number of output ports is determined by the number of index vectors, each specified as a separate vector entry in a cell array. Indices are 1-based and need not be unique.
      mask init:
      | [numOutports, flatLenVect, flatIdxVect] = dspblkmultiportsel(idxCellArray);
      mask Help: web(dspbhelp);
      mask StyleString: popup(Rows|Columns),edit,popup(Clip Index|Clip and Warn|Generate Error)
      mask Display: disp(['Select\n' &1]);
  Product2 : Product  Inputs=**  SaturateOnIntegerOverflow=on
  Product4 : Product  Inputs=/*  SaturateOnIntegerOverflow=on
  Transpose : dspmtrx3/Transpose  Hermitian=off  overflowFlag=on
  Transpose1 : dspmtrx3/Transpose  Hermitian=off  overflowFlag=on
  Transpose2 : dspmtrx3/Transpose  Hermitian=off  overflowFlag=on
  ch est : Outport
  wires:
  trn/1 -> Transpose/1
  Product4/1 -> Frame Status Conversion1/1
  Frame Status Conversion1/1 -> Transpose1/1
  Transpose1/1 -> ch est/1
  in/1 -> Transpose2/1
  Mean2/1 -> Enable Averaging/3
  Mean3/1 -> Enable Averaging1/3
  Transpose/1 -> Product2/1, Product2/2
  Transpose2/1 -> Mean3/1, One sym only (in)/1
  Product2/1 -> Mean2/1, One sym only (trn)/1
  Enable Averaging/1 -> Product4/1
  Nsts > 1/1 -> Enable Averaging/1, Enable Averaging1/1
  One sym only (in)/1 -> Enable Averaging1/2
  Enable Averaging1/1 -> Product4/2
  One sym only (trn)/1 -> Enable Averaging/2

== system ieee80211n/MIMODetection/Channel Estimation/ChannelEst5/Channel estimates ==
  trn : Inport  Port=1  LatchInput=off
  in : Inport  Port=2  LatchInput=off
  Enable Averaging : MultiPortSwitch  Inputs=2  zeroidx=on  SaturateOnIntegerOverflow=on
  Enable Averaging1 : MultiPortSwitch  Inputs=2  zeroidx=on  SaturateOnIntegerOverflow=on
  Frame Status Conversion1 : dspsigattribs/Frame Status Conversion  growRefPort=off  outframe=Frame-based
  Mean2 : dspstat3/Mean  DialogController=dspDDGCreate  DialogControllerArgs=DataTag25  run=off  reset_popup=None  roundingMode=Floor  overflowMode=off
  Mean3 : dspstat3/Mean  DialogController=dspDDGCreate  DialogControllerArgs=DataTag26  run=off  reset_popup=None  roundingMode=Floor  overflowMode=off
  Nsts > 1 : Constant  Value=params.NSTS > 1
  One sym only (in) : S-Function  AncestorBlock=dspindex/Multiport Selector  FunctionName=sdspmultiportsel  Parameters=rowsOrCols, numOutports, flatIdxVect, flatLenVect, idxErrMode  mask(Multiport Selector){rowsOrCols=Rows, idxCellArray=1, idxErrMode=Clip Index}
      mask prompts: rowsOrCols "Select:"; idxCellArray "Indices to output:"; idxErrMode "Invalid index:"
      mask help: Output specified rows or columns to one or more output ports. The number of output ports is determined by the number of index vectors, each specified as a separate vector entry in a cell array. Indices are 1-based and need not be unique.
      mask init:
      | [numOutports, flatLenVect, flatIdxVect] = dspblkmultiportsel(idxCellArray);
      mask Help: web(dspbhelp);
      mask StyleString: popup(Rows|Columns),edit,popup(Clip Index|Clip and Warn|Generate Error)
      mask Display: disp(['Select\n' &1]);
  One sym only (trn) : S-Function  AncestorBlock=dspindex/Multiport Selector  FunctionName=sdspmultiportsel  Parameters=rowsOrCols, numOutports, flatIdxVect, flatLenVect, idxErrMode  mask(Multiport Selector){rowsOrCols=Rows, idxCellArray=1, idxErrMode=Clip Index}
      mask prompts: rowsOrCols "Select:"; idxCellArray "Indices to output:"; idxErrMode "Invalid index:"
      mask help: Output specified rows or columns to one or more output ports. The number of output ports is determined by the number of index vectors, each specified as a separate vector entry in a cell array. Indices are 1-based and need not be unique.
      mask init:
      | [numOutports, flatLenVect, flatIdxVect] = dspblkmultiportsel(idxCellArray);
      mask Help: web(dspbhelp);
      mask StyleString: popup(Rows|Columns),edit,popup(Clip Index|Clip and Warn|Generate Error)
      mask Display: disp(['Select\n' &1]);
  Product2 : Product  Inputs=**  SaturateOnIntegerOverflow=on
  Product4 : Product  Inputs=/*  SaturateOnIntegerOverflow=on
  Transpose : dspmtrx3/Transpose  Hermitian=off  overflowFlag=on
  Transpose1 : dspmtrx3/Transpose  Hermitian=off  overflowFlag=on
  Transpose2 : dspmtrx3/Transpose  Hermitian=off  overflowFlag=on
  ch est : Outport
  wires:
  trn/1 -> Transpose/1
  Product4/1 -> Frame Status Conversion1/1
  Frame Status Conversion1/1 -> Transpose1/1
  Transpose1/1 -> ch est/1
  in/1 -> Transpose2/1
  Mean2/1 -> Enable Averaging/3
  Mean3/1 -> Enable Averaging1/3
  Transpose/1 -> Product2/1, Product2/2
  Transpose2/1 -> Mean3/1, One sym only (in)/1
  Product2/1 -> Mean2/1, One sym only (trn)/1
  Enable Averaging/1 -> Product4/1
  Nsts > 1/1 -> Enable Averaging/1, Enable Averaging1/1
  One sym only (in)/1 -> Enable Averaging1/2
  Enable Averaging1/1 -> Product4/2
  One sym only (trn)/1 -> Enable Averaging/2
